simulink model "s_opmdl"  (Simulink 4.00)
settings: Solver=ode45  SolverMode=SingleTasking  StartTime=0.0  StopTime=999999  MaxStep=10  RelTol=1e-3  AbsTol=1e-6
settings Model: LastModifiedBy=Administrator  SaveTime=off  SaveOutput=off  LimitDataPoints=off  BlockReductionOpt=off

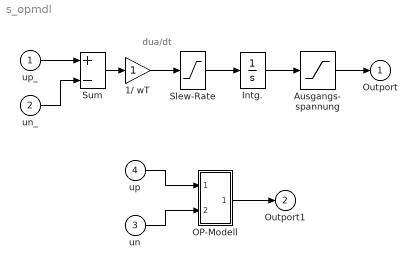
== system s_opmdl ==
  note: dua/dt
  up_ : Inport  Port=1
  un_ : Inport  Port=2
  un : Inport  Port=3
  up : Inport  Port=4
  1/ wT : Gain  Gain=1  Multiplication=Element-wise(K.*u)  SaturateOnIntegerOverflow=on
  Ausgangs- spannung : Saturate  UpperLimit=0.5  LowerLimit=-0.5  LinearizeAsGain=on
  Intg. : Integrator  ExternalReset=none  InitialConditionSource=internal  InitialCondition=0  LimitOutput=off  UpperSaturationLimit=inf  LowerSaturationLimit=-inf  ShowSaturationPort=off  ShowStatePort=off  AbsoluteTolerance=auto
  OP-Modell : Subsystem
      settings: RTWFcnNameOpts=Auto  RTWFileNameOpts=Auto
  Slew-Rate : Saturate  UpperLimit=0.5  LowerLimit=-0.5  LinearizeAsGain=on
  Sum : Sum  Inputs=+-  SaturateOnIntegerOverflow=on
  Outport : Outport  Port=1
  Outport1 : Outport  Port=2
  wires:
  OP-Modell/1(out_1) -> Outport1/1
  un/1 -> OP-Modell/2(in_2)
  up/1 -> OP-Modell/1(in_1)
  Ausgangs- spannung/1 -> Outport/1
  Intg./1 -> Ausgangs- spannung/1
  Slew-Rate/1 -> Intg./1
  1/ wT/1 -> Slew-Rate/1
  Sum/1 -> 1/ wT/1
  un_/1 -> Sum/2
  up_/1 -> Sum/1

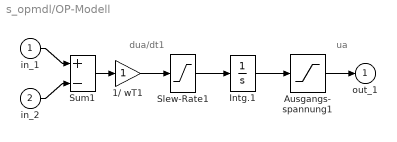
== system s_opmdl/OP-Modell ==
  note: dua/dt1
  note: ua
  in_1 : Inport  Port=1
  in_2 : Inport  Port=2
  1/ wT1 : Gain  Gain=1  Multiplication=Element-wise(K.*u)  SaturateOnIntegerOverflow=on
  Ausgangs- spannung1 : Saturate  UpperLimit=0.5  LowerLimit=-0.5  LinearizeAsGain=on
  Intg.1 : Integrator  ExternalReset=none  InitialConditionSource=internal  InitialCondition=0  LimitOutput=off  UpperSaturationLimit=inf  LowerSaturationLimit=-inf  ShowSaturationPort=off  ShowStatePort=off  AbsoluteTolerance=auto
  Slew-Rate1 : Saturate  UpperLimit=0.5  LowerLimit=-0.5  LinearizeAsGain=on
  Sum1 : Sum  Inputs=+-  SaturateOnIntegerOverflow=on
  out_1 : Outport  Port=1
  wires:
  in_2/1 -> Sum1/2
  Ausgangs- spannung1/1 -> out_1/1
  in_1/1 -> Sum1/1
  Sum1/1 -> 1/ wT1/1
  1/ wT1/1 -> Slew-Rate1/1
  Slew-Rate1/1 -> Intg.1/1
  Intg.1/1 -> Ausgangs- spannung1/1
